simulink model "feedback"  (R2016b)
settings: Solver=VariableStepAuto  StartTime=0.0  StopTime=inf  RelTol=1e-3
libraries: dspvision x3, dspsnks4 x1
settings Model: Creator=91243  LastModifiedBy=91243

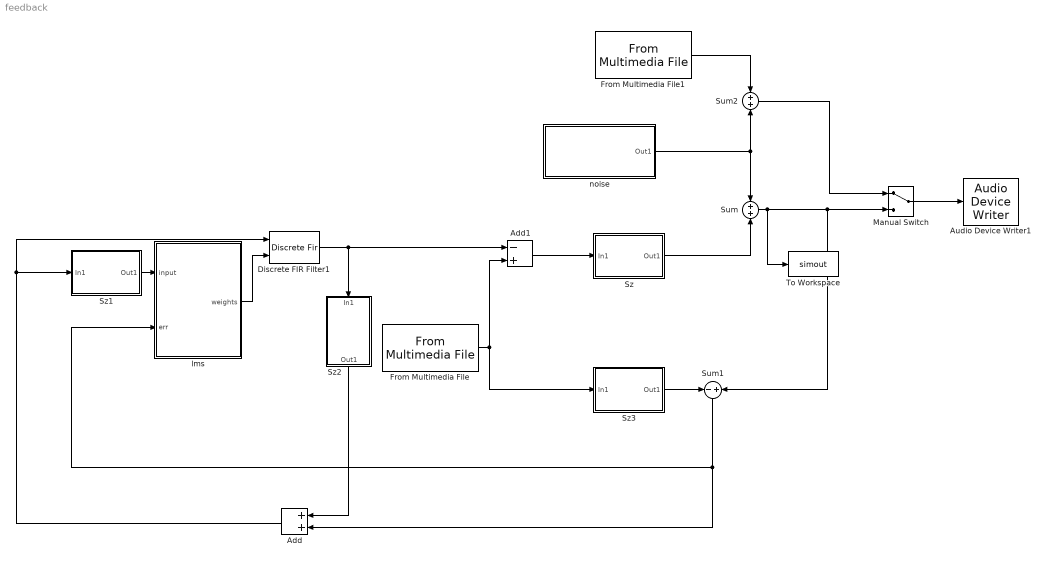
== system feedback ==
  Add : Sum
  Add1 : Sum  Inputs=-+
  Audio Device Writer1 : dspsnks4/Audio Device Writer  Driver=DirectSound  Device=Default  InheritSampleRate=off  SampleRate=8192  BitDepth=16-bit integer  BufferSize=4096  NumBuffers=10  DefaultOutputChannelMapping=on  OutputChannelMapping=1:2  OutputNumUnderrunSamples=off  DriverIdx=1  DeviceWarnFlag=''
  Discrete FIR Filter1 : DiscreteFir  CoefSource=Input port  Coefficients=[0.5 0.5 0.3 0.3]
      settings: InputPortMap=u0,u1
  From Multimedia File : dspvision/From Multimedia File  inputFilename=C:\Users\91243\Downloads\lab\project\codes\Music.wav  loop=on  numPlays=inf  outputStreams=Audio only  videoDataType=single  audioDataType=double  inheritSampleTime=on  userDefinedSampleTime=1/10  noAudioOutput=off  isIntensityVideo=off  fourcc=RGB  colorVideoFormat=Separate color signals  outputEOF=off  dataOrg=Column-major  audioFrameSize=512  computeAudioFrameSize=off  outSamplingMode=Sample based
  From Multimedia File1 : dspvision/From Multimedia File  inputFilename=C:\Users\91243\Downloads\lab\project\codes\Music.wav  loop=on  numPlays=inf  outputStreams=Audio only  videoDataType=single  audioDataType=double  inheritSampleTime=on  userDefinedSampleTime=1/30  noAudioOutput=off  isIntensityVideo=off  fourcc=RGB  colorVideoFormat=Separate color signals  outputEOF=off  dataOrg=Column-major  audioFrameSize=512  computeAudioFrameSize=off  outSamplingMode=Sample based
  Manual Switch : ManualSwitch
  Sum : Sum
  Sum1 : Sum  Inputs=-+
  Sum2 : Sum
  Sz : Subsystem
  Sz1 : Subsystem
  Sz2 : Subsystem
  Sz3 : Subsystem
  To Workspace : ToWorkspace  VariableName=simout  SaveFormat=Timeseries  SampleTime=-1
  lms : Subsystem
  noise : Subsystem
  wires:
  Sz/1(Out1) -> Sum/2
  noise/1(Out1) -> Sum/1, Sum2/2
  Sz2/1(Out1) -> Add/1
  Discrete FIR Filter1/1 -> Add1/1, Sz2/1(In1)
  Add/1 -> Sz1/1(In1), Discrete FIR Filter1/1
  Sum/1 -> To Workspace/1, Sum1/2, Manual Switch/2
  Manual Switch/1 -> Audio Device Writer1/1
  Sz1/1(Out1) -> lms/1("input ")
  lms/1("weights ") -> Discrete FIR Filter1/2
  From Multimedia File/1 -> Add1/2, Sz3/1(In1)
  Add1/1 -> Sz/1(In1)
  Sz3/1(Out1) -> Sum1/1
  Sum1/1 -> lms/2(err), Add/2
  From Multimedia File1/1 -> Sum2/1
  Sum2/1 -> Manual Switch/1

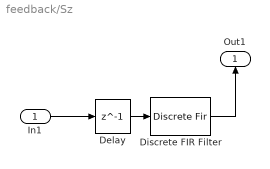
== system feedback/Sz ==
  In1 : Inport
  Delay : Delay  DelayLength=1  InitialCondition=0
  Discrete FIR Filter : DiscreteFir  Coefficients=[0.5 0.5 0.3 0.3]
  Out1 : Outport
  wires:
  In1/1 -> Delay/1
  Delay/1 -> Discrete FIR Filter/1
  Discrete FIR Filter/1 -> Out1/1

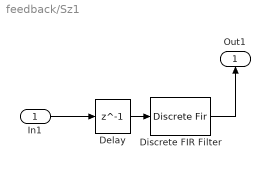
== system feedback/Sz1 ==
  In1 : Inport
  Delay : Delay  DelayLength=1  InitialCondition=0
  Discrete FIR Filter : DiscreteFir  Coefficients=[0.5 0.5 0.3 0.3]
  Out1 : Outport
  wires:
  In1/1 -> Delay/1
  Delay/1 -> Discrete FIR Filter/1
  Discrete FIR Filter/1 -> Out1/1

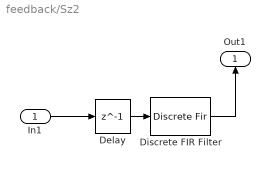
== system feedback/Sz2 ==
  In1 : Inport
  Delay : Delay  DelayLength=1  InitialCondition=0
  Discrete FIR Filter : DiscreteFir  Coefficients=[0.5 0.5 0.3 0.3]
  Out1 : Outport
  wires:
  In1/1 -> Delay/1
  Delay/1 -> Discrete FIR Filter/1
  Discrete FIR Filter/1 -> Out1/1

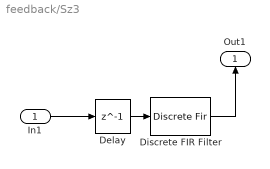
== system feedback/Sz3 ==
  In1 : Inport
  Delay : Delay  DelayLength=1  InitialCondition=0
  Discrete FIR Filter : DiscreteFir  Coefficients=[0.5 0.5 0.3 0.3]
  Out1 : Outport
  wires:
  In1/1 -> Delay/1
  Delay/1 -> Discrete FIR Filter/1
  Discrete FIR Filter/1 -> Out1/1

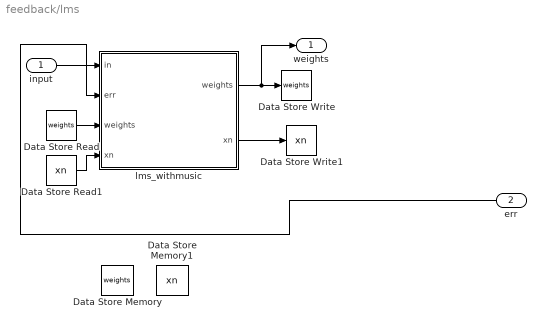
== system feedback/lms ==
  "input " : Inport
  err : Inport  Port=2
  Data Store Memory : DataStoreMemory  DataStoreName=weights  ReadBeforeWriteMsg=warning  WriteAfterWriteMsg=warning  WriteAfterReadMsg=warning  ShowAdditionalParam=off  Dimensions=256
  Data Store Memory1 : DataStoreMemory  DataStoreName=xn  ReadBeforeWriteMsg=warning  WriteAfterWriteMsg=warning  WriteAfterReadMsg=warning  ShowAdditionalParam=off  Dimensions=256
  Data Store Read : DataStoreRead  DataStoreName=weights
  Data Store Read1 : DataStoreRead  DataStoreName=xn
  Data Store Write : DataStoreWrite  DataStoreName=weights
  Data Store Write1 : DataStoreWrite  DataStoreName=xn
  lms_withmusic : MATLAB Function  TreatAsAtomicUnit=on
  "weights " : Outport
  wires:
  lms_withmusic/2(xn) -> Data Store Write1/1
  Data Store Read/1 -> lms_withmusic/3("weights ")
  Data Store Read1/1 -> lms_withmusic/4("xn ")
  lms_withmusic/1(weights) -> "weights "/1, Data Store Write/1
  "input "/1 -> lms_withmusic/1(in)
  err/1 -> lms_withmusic/2(err)

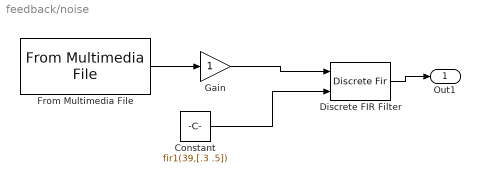
== system feedback/noise ==
  Constant : Constant  Value=fir1(39,[.3 .5])
  Discrete FIR Filter : DiscreteFir  CoefSource=Input port
      settings: InputPortMap=u0,u1
  From Multimedia File : dspvision/From Multimedia File  inputFilename=C:\Users\91243\Downloads\lab\project\codes\Noise.wav  loop=on  numPlays=inf  outputStreams=Audio only  videoDataType=single  audioDataType=double  inheritSampleTime=on  userDefinedSampleTime=1/44.1  noAudioOutput=off  isIntensityVideo=off  fourcc=RGB  colorVideoFormat=Separate color signals  outputEOF=off  dataOrg=Column-major  audioFrameSize=512  computeAudioFrameSize=off  outSamplingMode=Sample based
  Gain : Gain
  Out1 : Outport
  wires:
  From Multimedia File/1 -> Gain/1
  Constant/1 -> Discrete FIR Filter/2
  Gain/1 -> Discrete FIR Filter/1
  Discrete FIR Filter/1 -> Out1/1

== matlab function feedback/lms/lms_withmusic ==
  data: in input; weights output; err input; weights input; xn input; xn output
function [weights,xn] = func_withmu(in,err,weights,xn)
    testing = in;
    length = 256;
    %mu = 0.1;
    mu = 0.0001;
    xn = [ sum(in); xn(1:length-1,1)];
    weights = weights+ mu*xn*sum(err);
    %weights = weights+ mu/norm(xn,2)*xn*sum(err);
end
